simulink library "ifo_new"  (Simulink 8.1)
settings: Solver=ode45  StartTime=0.0  StopTime=10.0  RelTol=1e-3
libraries: hmi x1, gaps x1, ttc x1, sft x1, veh x1, veh_new x1
settings Model: Creator=xsellart  LastModifiedBy=tescamilla

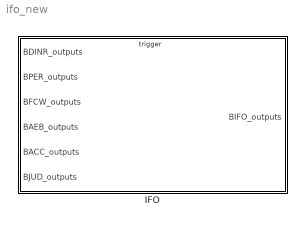
== system ifo_new ==
  IFO : Subsystem

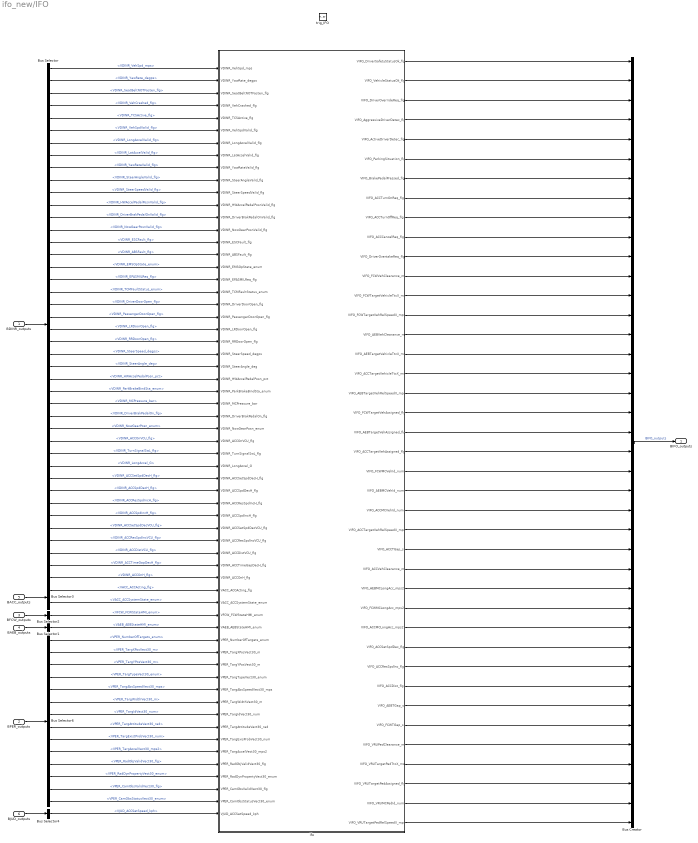
== system ifo_new/IFO ==
  BDINR_outputs : Inport  OutDataTypeStr=Bus: BDINR_outputs
  BPER_outputs : Inport  Port=2  OutDataTypeStr=Bus: BPER_outputs
  BFCW_outputs : Inport  Port=3  OutDataTypeStr=Bus: BFCW_outputs
  BAEB_outputs : Inport  Port=4  OutDataTypeStr=Bus: BAEB_outputs
  BACC_outputs : Inport  Port=5  OutDataTypeStr=Bus: BACC_outputs
  BJUD_outputs : Inport  Port=6  OutDataTypeStr=Bus: BJUD_outputs
  trig_IFO : TriggerPort  TriggerType=function-call
      settings: AttributesFormatString=State = %<StatesWhenEnabling>
  Bus Creator : BusCreator  Inputs=40  OutDataTypeStr=Bus: BIFO_outputs
  Bus Selector : BusSelector  OutputSignals=VDINR_VehSpd_mps,VDINR_YawRate_degps,VDINR_SeatBeltNOTFasten_flg,VDINR_VehCrashed_flg,VDINR_TCSActive_flg,VDINR_VehSpdValid_flg,VDINR_LongAccelValid_flg,VDINR_LatAccelValid_flg,VDINR_YawRateValid_flg,VDINR_SteerAngleValid_flg,VDINR_SteerSpeedValid_flg,VDINR_HWAccelPedalPosnValid_flg,VDINR_DriverBrakPedalOnValid_flg,VDINR_NowGearPosnValid_flg,VDINR_ESCFault_flg,VDINR_ABSFault_flg,VDINR_EMSOpState_enum,VDINR_EPASMILReq_flg,VDINR_TCMFaultStatus_enum,VDINR_DriverDoorOpen_flg,VDINR_PassengerDoorOpen_flg,VDINR_LRDoorOpen_flg,VDINR_RRDoorOpen_flg,VDINR_SteerSpeed_degps,VDINR_SteerAngle_deg,VDINR_HWAccelPedalPosn_pct,VDINR_ParkBrakeBindSta_enum,VDINR_MCPressure_bar,VDINR_DriverBrakPedalOn_flg,VDINR_NowGearPosn_enum,VDINR_ACCOnVCU_flg,VDINR_TurnSignalSwL_flg,VDINR_LongAccel_G,VDINR_ACCSetSpdDecH_flg,VDINR_ACCSpdDecH_flg,VDINR_ACCResSpdIncH_flg,VDINR_ACCSpdIncH_flg,VDINR_ACCSetSpdDecVCU_flg,VDINR_ACCResSpdIncVCU_flg,VDINR_ACCDistVCU_flg,VDINR_ACCTimeGapDecH_flg,VDINR_ACCOnH_flg
  Bus Selector1 : BusSelector  OutputSignals=VAEB_AEBStateHMI_enum
  Bus Selector2 : BusSelector  OutputSignals=VFCW_FCWStateHMI_enum
  Bus Selector3 : BusSelector  OutputSignals=VACC_ACCActing_flg,VACC_ACCSystemState_enum
  Bus Selector4 : BusSelector  OutputSignals=VJUD_ACCSetSpeed_kph
  Bus Selector6 : BusSelector  OutputSignals=VPER_NumberOfTargets_enum,VPER_TargXPosVect30_m,VPER_TargYPosVect30_m,VPER_TargTypeVect30_enum,VPER_TargAbsSpeedVect30_mps,VPER_TargWidthVect30_m,VPER_TargIdVect30_num,VPER_TargAttitudeVect30_rad,VPER_TargExistProbVect30_num,VPER_TargAccelVect30_mps2,VPER_RadObjValidVect30_flg,VPER_RadDynPropertyVect30_enum,VPER_CamObsValidVect30_flg,VPER_CamObsStatusVect30_enum
  ifo : Subsystem
  BIFO_outputs : Outport  OutDataTypeStr=Bus: BIFO_outputs
  wires:
  ifo/26(VIFO_ACCTGap_s) -> Bus Creator/26
  ifo/25(VIFO_ACCTargetVehRelSpeedX_mps) -> Bus Creator/25
  ifo/24(VIFO_ACCMCVehId_num) -> Bus Creator/24
  ifo/23(VIFO_AEBMCVehId_num) -> Bus Creator/23
  ifo/22(VIFO_FCWMCVehId_num) -> Bus Creator/22
  ifo/20(VIFO_AEBTargetVehAssigned_flg) -> Bus Creator/20
  ifo/18(VIFO_AEBTargetVehRelSpeedX_mps) -> Bus Creator/18
  ifo/16(VIFO_AEBTargetVehicleTtcX_ms) -> Bus Creator/16
  ifo/15(VIFO_AEBVehClearance_m) -> Bus Creator/15
  ifo/14(VIFO_FCWTargetVehRelSpeedX_mps) -> Bus Creator/14
  ifo/13(VIFO_FCWTargetVehicleTtcX_ms) -> Bus Creator/13
  ifo/12(VIFO_FCWVehClearance_m) -> Bus Creator/12
  ifo/10(VIFO_ACCCancelReq_flg) -> Bus Creator/10
  ifo/8(VIFO_ACCTurnOnReq_flg) -> Bus Creator/8
  ifo/9(VIFO_ACCTurnOffReq_flg) -> Bus Creator/9
  BDINR_outputs/1 -> Bus Selector/1
  BFCW_outputs/1 -> Bus Selector2/1
  BPER_outputs/1 -> Bus Selector6/1
  Bus Creator/1 -> BIFO_outputs/1  "BIFO_outputs"
  ifo/5(VIFO_ActiveDriverDetec_flg) -> Bus Creator/5
  ifo/4(VIFO_AggressiveDriverDetec_flg) -> Bus Creator/4
  ifo/7(VIFO_BrakePedalPressed_flg) -> Bus Creator/7
  ifo/6(VIFO_ParkingSituation_flg) -> Bus Creator/6
  ifo/1(VIFO_DriverSafetyStatusOk_flg) -> Bus Creator/1
  ifo/3(VIFO_DriverOverrideReq_flg) -> Bus Creator/3
  ifo/2(VIFO_VehicleStatusOk_flg) -> Bus Creator/2
  BAEB_outputs/1 -> Bus Selector1/1
  ifo/27(VIFO_ACCVehClearance_m) -> Bus Creator/27
  ifo/11(VIFO_DriverOvertakeReq_flg) -> Bus Creator/11
  Bus Selector/19 -> ifo/19(VDINR_TCMFaultStatus_enum)  "<VDINR_TCMFaultStatus_enum>"
  Bus Selector/21 -> ifo/21(VDINR_PassengerDoorOpen_flg)  "<VDINR_PassengerDoorOpen_flg>"
  Bus Selector/13 -> ifo/13(VDINR_DriverBrakPedalOnValid_flg)  "<VDINR_DriverBrakPedalOnValid_flg>"
  Bus Selector/11 -> ifo/11(VDINR_SteerSpeedValid_flg)  "<VDINR_SteerSpeedValid_flg>"
  Bus Selector/17 -> ifo/17(VDINR_EMSOpState_enum)  "<VDINR_EMSOpState_enum>"
  Bus Selector/12 -> ifo/12(VDINR_HWAccelPedalPosnValid_flg)  "<VDINR_HWAccelPedalPosnValid_flg>"
  Bus Selector/14 -> ifo/14(VDINR_NowGearPosnValid_flg)  "<VDINR_NowGearPosnValid_flg>"
  Bus Selector/18 -> ifo/18(VDINR_EPASMILReq_flg)  "<VDINR_EPASMILReq_flg>"
  Bus Selector/16 -> ifo/16(VDINR_ABSFault_flg)  "<VDINR_ABSFault_flg>"
  Bus Selector/8 -> ifo/8(VDINR_LatAccelValid_flg)  "<VDINR_LatAccelValid_flg>"
  Bus Selector/20 -> ifo/20(VDINR_DriverDoorOpen_flg)  "<VDINR_DriverDoorOpen_flg>"
  Bus Selector/9 -> ifo/9(VDINR_YawRateValid_flg)  "<VDINR_YawRateValid_flg>"
  Bus Selector/15 -> ifo/15(VDINR_ESCFault_flg)  "<VDINR_ESCFault_flg>"
  Bus Selector/10 -> ifo/10(VDINR_SteerAngleValid_flg)  "<VDINR_SteerAngleValid_flg>"
  Bus Selector/22 -> ifo/22(VDINR_LRDoorOpen_flg)  "<VDINR_LRDoorOpen_flg>"
  Bus Selector/23 -> ifo/23(VDINR_RRDoorOpen_flg)  "<VDINR_RRDoorOpen_flg>"
  Bus Selector/3 -> ifo/3(VDINR_SeatBeltNOTFasten_flg)  "<VDINR_SeatBeltNOTFasten_flg>"
  Bus Selector/6 -> ifo/6(VDINR_VehSpdValid_flg)  "<VDINR_VehSpdValid_flg>"
  Bus Selector/24 -> ifo/24(VDINR_SteerSpeed_degps)  "<VDINR_SteerSpeed_degps>"
  Bus Selector/2 -> ifo/2(VDINR_YawRate_degps)  "<VDINR_YawRate_degps>"
  Bus Selector/4 -> ifo/4(VDINR_VehCrashed_flg)  "<VDINR_VehCrashed_flg>"
  Bus Selector/1 -> ifo/1(VDINR_VehSpd_mps)  "<VDINR_VehSpd_mps>"
  Bus Selector/7 -> ifo/7(VDINR_LongAccelValid_flg)  "<VDINR_LongAccelValid_flg>"
  Bus Selector/5 -> ifo/5(VDINR_TCSActive_flg)  "<VDINR_TCSActive_flg>"
  Bus Selector/30 -> ifo/30(VDINR_NowGearPosn_enum)  "<VDINR_NowGearPosn_enum>"
  Bus Selector/29 -> ifo/29(VDINR_DriverBrakPedalOn_flg)  "<VDINR_DriverBrakPedalOn_flg>"
  Bus Selector/28 -> ifo/28(VDINR_MCPressure_bar)  "<VDINR_MCPressure_bar>"
  Bus Selector/27 -> ifo/27(VDINR_ParkBrakeBindSta_enum)  "<VDINR_ParkBrakeBindSta_enum>"
  Bus Selector/26 -> ifo/26(VDINR_HWAccelPedalPosn_pct)  "<VDINR_HWAccelPedalPosn_pct>"
  Bus Selector/25 -> ifo/25(VDINR_SteerAngle_deg)  "<VDINR_SteerAngle_deg>"
  BACC_outputs/1 -> Bus Selector3/1
  Bus Selector1/1 -> ifo/46(VAEB_AEBStateHMI_enum)  "<VAEB_AEBStateHMI_enum>"
  Bus Selector2/1 -> ifo/45(VFCW_FCWStateHMI_enum)  "<VFCW_FCWStateHMI_enum>"
  Bus Selector3/1 -> ifo/43(VACC_ACCActing_flg)  "<VACC_ACCActing_flg>"
  Bus Selector3/2 -> ifo/44(VACC_ACCSystemState_enum)  "<VACC_ACCSystemState_enum>"
  Bus Selector/32 -> ifo/32(VDINR_TurnSignalSwL_flg)  "<VDINR_TurnSignalSwL_flg>"
  Bus Selector6/1 -> ifo/47(VPER_NumberOfTargets_enum)  "<VPER_NumberOfTargets_enum>"
  Bus Selector6/2 -> ifo/48(VPER_TargXPosVect30_m)  "<VPER_TargXPosVect30_m>"
  Bus Selector6/3 -> ifo/49(VPER_TargYPosVect30_m)  "<VPER_TargYPosVect30_m>"
  Bus Selector6/4 -> ifo/50(VPER_TargTypeVect30_enum)  "<VPER_TargTypeVect30_enum>"
  Bus Selector6/9 -> ifo/55(VPER_TargExisProbVect30_num)  "<VPER_TargExistProbVect30_num>"
  Bus Selector6/6 -> ifo/52(VPER_TargWidthVect30_m)  "<VPER_TargWidthVect30_m>"
  Bus Selector6/7 -> ifo/53(VPER_TargIdVect30_num)  "<VPER_TargIdVect30_num>"
  Bus Selector6/8 -> ifo/54(VPER_TargAttitudeVect30_rad)  "<VPER_TargAttitudeVect30_rad>"
  Bus Selector6/5 -> ifo/51(VPER_TargAbsSpeedVect30_mps)  "<VPER_TargAbsSpeedVect30_mps>"
  BJUD_outputs/1 -> Bus Selector4/1
  Bus Selector4/1 -> ifo/61(VJUD_ACCSetSpeed_kph)  "<VJUD_ACCSetSpeed_kph>"
  Bus Selector/31 -> ifo/31(VDINR_ACCOnVCU_flg)  "<VDINR_ACCOnVCU_flg>"
  Bus Selector/33 -> ifo/33(VDINR_LongAccel_G)  "<VDINR_LongAccel_G>"
  ifo/28(VIFO_AEBMCLongAcc_mps2) -> Bus Creator/28
  ifo/30(VIFO_ACCMCLongAcc_mps2) -> Bus Creator/30
  ifo/29(VIFO_FCWMCLongAcc_mps2) -> Bus Creator/29
  Bus Selector6/11 -> ifo/57(VPER_RadObjValidVect30_flg)  "<VPER_RadObjValidVect30_flg>"
  Bus Selector6/12 -> ifo/58(VPER_RadDynPropertyVect30_enum)  "<VPER_RadDynPropertyVect30_enum>"
  Bus Selector6/10 -> ifo/56(VPER_TargAccelVect30_mps2)  "<VPER_TargAccelVect30_mps2>"
  Bus Selector6/14 -> ifo/60(VPER_CamObsStatusVect30_enum)  "<VPER_CamObsStatusVect30_enum>"
  Bus Selector6/13 -> ifo/59(VPER_CamObsValidVect30_flg)  "<VPER_CamObsValidVect30_flg>"
  ifo/17(VIFO_ACCTargetVehicleTtcX_ms) -> Bus Creator/17
  ifo/21(VIFO_ACCTargetVehAssigned_flg) -> Bus Creator/21
  ifo/19(VIFO_FCWTargetVehAssigned_flg) -> Bus Creator/19
  ifo/32(VIFO_ACCResSpdInc_flg) -> Bus Creator/32
  ifo/33(VIFO_ACCDist_flg) -> Bus Creator/33
  ifo/31(VIFO_ACCSetSpdDec_flg) -> Bus Creator/31
  Bus Selector/34 -> ifo/34(VDINR_ACCSetSpdDecH_flg)  "<VDINR_ACCSetSpdDecH_flg>"
  Bus Selector/35 -> ifo/35(VDINR_ACCSpdDecH_flg)  "<VDINR_ACCSpdDecH_flg>"
  Bus Selector/36 -> ifo/36(VDINR_ACCResSpdIncH_flg)  "<VDINR_ACCResSpdIncH_flg>"
  Bus Selector/37 -> ifo/37(VDINR_ACCSpdIncH_flg)  "<VDINR_ACCSpdIncH_flg>"
  Bus Selector/39 -> ifo/39(VDINR_ACCResSpdIncVCU_flg)  "<VDINR_ACCResSpdIncVCU_flg>"
  Bus Selector/38 -> ifo/38(VDINR_ACCSetSpdDecVCU_flg)  "<VDINR_ACCSetSpdDecVCU_flg>"
  Bus Selector/42 -> ifo/42(VDINR_ACCOnH_flg)  "<VDINR_ACCOnH_flg>"
  Bus Selector/41 -> ifo/41(VDINR_ACCTimeGapDecH_flg)  "<VDINR_ACCTimeGapDecH_flg>"
  Bus Selector/40 -> ifo/40(VDINR_ACCDistVCU_flg)  "<VDINR_ACCDistVCU_flg>"
  ifo/34(VIFO_AEBTGap_s) -> Bus Creator/34
  ifo/35(VIFO_FCWTGap_s) -> Bus Creator/35
  ifo/38(VIFO_VRUTargetPedAssigned_flg) -> Bus Creator/38
  ifo/36(VIFO_VRUPedClearance_m) -> Bus Creator/36
  ifo/39(VIFO_VRUMCPedId_num) -> Bus Creator/39
  ifo/37(VIFO_VRUTargetPedTtcX_ms) -> Bus Creator/37
  ifo/40(VIFO_VRUTargetPedRelSpeedX_mps) -> Bus Creator/40

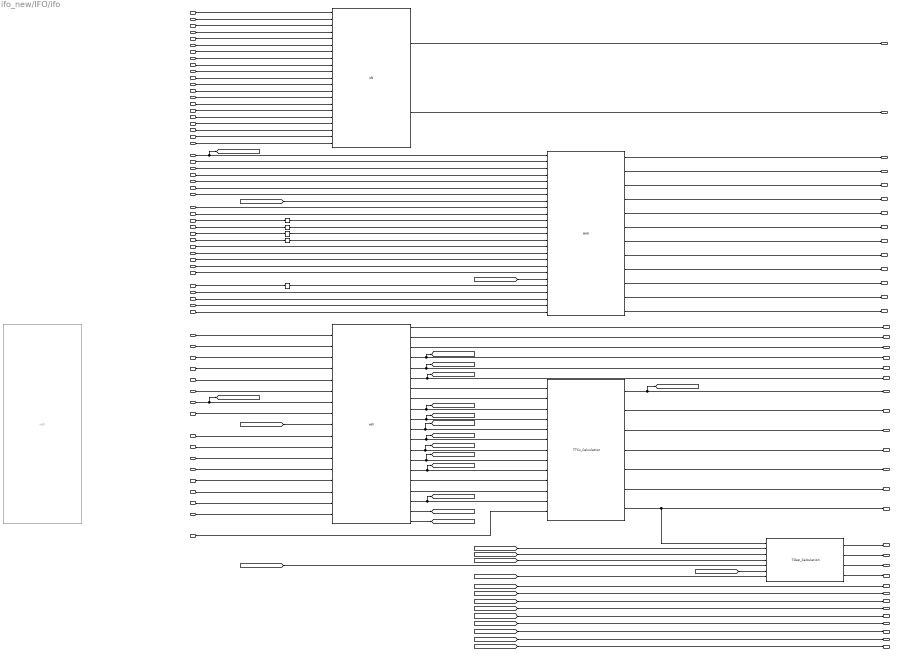
== system ifo_new/IFO/ifo ==
  VDINR_VehSpd_mps : Inport
  VDINR_YawRate_degps : Inport  Port=2
  VDINR_SeatBeltNOTFasten_flg : Inport  Port=3
  VDINR_VehCrashed_flg : Inport  Port=4
  VDINR_TCSActive_flg : Inport  Port=5
  VDINR_VehSpdValid_flg : Inport  Port=6
  VDINR_LongAccelValid_flg : Inport  Port=7
  VDINR_LatAccelValid_flg : Inport  Port=8
  VDINR_YawRateValid_flg : Inport  Port=9
  VDINR_SteerAngleValid_flg : Inport  Port=10
  VDINR_SteerSpeedValid_flg : Inport  Port=11
  VDINR_HWAccelPedalPosnValid_flg : Inport  Port=12
  VDINR_DriverBrakPedalOnValid_flg : Inport  Port=13
  VDINR_NowGearPosnValid_flg : Inport  Port=14
  VDINR_ESCFault_flg : Inport  Port=15
  VDINR_ABSFault_flg : Inport  Port=16
  VDINR_EMSOpState_enum : Inport  Port=17
  VDINR_EPASMILReq_flg : Inport  Port=18
  VDINR_TCMFaultStatus_enum : Inport  Port=19
  VDINR_DriverDoorOpen_flg : Inport  Port=20
  VDINR_PassengerDoorOpen_flg : Inport  Port=21
  VDINR_LRDoorOpen_flg : Inport  Port=22
  VDINR_RRDoorOpen_flg : Inport  Port=23
  VDINR_SteerSpeed_degps : Inport  Port=24
  VDINR_SteerAngle_deg : Inport  Port=25
  VDINR_HWAccelPedalPosn_pct : Inport  Port=26
  VDINR_ParkBrakeBindSta_enum : Inport  Port=27
  VDINR_MCPressure_bar : Inport  Port=28
  VDINR_DriverBrakPedalOn_flg : Inport  Port=29
  VDINR_NowGearPosn_enum : Inport  Port=30
  VDINR_ACCOnVCU_flg : Inport  Port=31
  VDINR_TurnSignalSwL_flg : Inport  Port=32
  VDINR_LongAccel_G : Inport  Port=33
  VDINR_ACCSetSpdDecH_flg : Inport  Port=34
  VDINR_ACCSpdDecH_flg : Inport  Port=35
  VDINR_ACCResSpdIncH_flg : Inport  Port=36
  VDINR_ACCSpdIncH_flg : Inport  Port=37
  VDINR_ACCSetSpdDecVCU_flg : Inport  Port=38
  VDINR_ACCResSpdIncVCU_flg : Inport  Port=39
  VDINR_ACCDistVCU_flg : Inport  Port=40
  VDINR_ACCTimeGapDecH_flg : Inport  Port=41
  VDINR_ACCOnH_flg : Inport  Port=42
  VACC_ACCActing_flg : Inport  Port=43
  VACC_ACCSystemState_enum : Inport  Port=44
  VFCW_FCWStateHMI_enum : Inport  Port=45
  VAEB_AEBStateHMI_enum : Inport  Port=46
  VPER_NumberOfTargets_enum : Inport  Port=47
  VPER_TargXPosVect30_m : Inport  Port=48
  VPER_TargYPosVect30_m : Inport  Port=49
  VPER_TargTypeVect30_enum : Inport  Port=50
  VPER_TargAbsSpeedVect30_mps : Inport  Port=51
  VPER_TargWidthVect30_m : Inport  Port=52
  VPER_TargIdVect30_num : Inport  Port=53
  VPER_TargAttitudeVect30_rad : Inport  Port=54
  VPER_TargExisProbVect30_num : Inport  Port=55
  VPER_TargAccelVect30_mps2 : Inport  Port=56
  VPER_RadObjValidVect30_flg : Inport  Port=57
  VPER_RadDynPropertyVect30_enum : Inport  Port=58
  VPER_CamObsValidVect30_flg : Inport  Port=59
  VPER_CamObsStatusVect30_enum : Inport  Port=60
  VJUD_ACCSetSpeed_kph : Inport  Port=61
  Delay{,1..4} (5 alike) : Delay  DelayLength=1  InitialCondition=0
  HMI : hmi/HMI
  TGap_Calculation : gaps/TGap_Calculation
  TTCx_Calculation : ttc/TTCx_Calculation
  sft : sft/sft
  veh : veh/veh  Commented=on
  veh1 : veh_new/veh
  VIFO_DriverSafetyStatusOk_flg : Outport
  VIFO_VehicleStatusOk_flg : Outport  Port=2
  VIFO_DriverOverrideReq_flg : Outport  Port=3
  VIFO_AggressiveDriverDetec_flg : Outport  Port=4
  VIFO_ActiveDriverDetec_flg : Outport  Port=5
  VIFO_ParkingSituation_flg : Outport  Port=6
  VIFO_BrakePedalPressed_flg : Outport  Port=7
  VIFO_ACCTurnOnReq_flg : Outport  Port=8
  VIFO_ACCTurnOffReq_flg : Outport  Port=9
  VIFO_ACCCancelReq_flg : Outport  Port=10
  VIFO_DriverOvertakeReq_flg : Outport  Port=11
  VIFO_FCWVehClearance_m : Outport  Port=12
  VIFO_FCWTargetVehicleTtcX_ms : Outport  Port=13
  VIFO_FCWTargetVehRelSpeedX_mps : Outport  Port=14
  VIFO_AEBVehClearance_m : Outport  Port=15
  VIFO_AEBTargetVehicleTtcX_ms : Outport  Port=16
  VIFO_ACCTargetVehicleTtcX_ms : Outport  Port=17
  VIFO_AEBTargetVehRelSpeedX_mps : Outport  Port=18
  VIFO_FCWTargetVehAssigned_flg : Outport  Port=19
  VIFO_AEBTargetVehAssigned_flg : Outport  Port=20
  VIFO_ACCTargetVehAssigned_flg : Outport  Port=21
  VIFO_FCWMCVehId_num : Outport  Port=22
  VIFO_AEBMCVehId_num : Outport  Port=23
  VIFO_ACCMCVehId_num : Outport  Port=24
  VIFO_ACCTargetVehRelSpeedX_mps : Outport  Port=25
  VIFO_ACCTGap_s : Outport  Port=26
  VIFO_ACCVehClearance_m : Outport  Port=27
  VIFO_AEBMCLongAcc_mps2 : Outport  Port=28
  VIFO_FCWMCLongAcc_mps2 : Outport  Port=29
  VIFO_ACCMCLongAcc_mps2 : Outport  Port=30
  VIFO_ACCSetSpdDec_flg : Outport  Port=31
  VIFO_ACCResSpdInc_flg : Outport  Port=32
  VIFO_ACCDist_flg : Outport  Port=33
  VIFO_AEBTGap_s : Outport  Port=34
  VIFO_FCWTGap_s : Outport  Port=35
  VIFO_VRUPedClearance_m : Outport  Port=36
  VIFO_VRUTargetPedTtcX_ms : Outport  Port=37
  VIFO_VRUTargetPedAssigned_flg : Outport  Port=38
  VIFO_VRUMCPedId_num : Outport  Port=39
  VIFO_VRUTargetPedRelSpeedX_mps : Outport  Port=40
  wires:
  [VIFO_ACCMCLongAcc_mps2] -> VIFO_ACCMCLongAcc_mps2/1
  [VIFO_ACCTargetVehRelSpeedX_mps] -> VIFO_ACCTargetVehRelSpeedX_mps/1
  veh1/6 -> VIFO_ACCTargetVehAssigned_flg/1, [VIFO_ACCTargetVehAssigned_flg]
  veh1/5 -> VIFO_AEBTargetVehAssigned_flg/1, [VIFO_AEBTargetVehAssigned_flg]
  veh1/4 -> VIFO_FCWTargetVehAssigned_flg/1, [VIFO_FCWTargetVehAssigned_flg]
  veh1/7 -> TTCx_Calculation/1
  veh1/8 -> TTCx_Calculation/2
  veh1/9 -> [VIFO_ACCMCVehXPosition_m], TTCx_Calculation/3
  veh1/10 -> [VIFO_FCWTargetVehRelSpeedX_mps], TTCx_Calculation/4
  veh1/11 -> TTCx_Calculation/5, [VIFO_AEBTargetVehRelSpeedX_mps]
  veh1/12 -> [VIFO_ACCTargetVehRelSpeedX_mps], TTCx_Calculation/6
  veh1/13 -> [VIFO_FCWMCLongAcc_mps2], TTCx_Calculation/7
  veh1/14 -> TTCx_Calculation/8, [VIFO_AEBMCLongAcc_mps2]
  veh1/15 -> [VIFO_ACCMCLongAcc_mps2], TTCx_Calculation/9
  TGap_Calculation/3 -> VIFO_AEBTGap_s/1
  TGap_Calculation/2 -> VIFO_ACCTGap_s/1
  [VDINR_VehSpd_mps] -> TGap_Calculation/5
  [VDINR_VehSpd_mps] -> HMI/8
  HMI/7 -> VIFO_ACCTurnOffReq_flg/1
  veh1/2 -> VIFO_AEBMCVehId_num/1
  veh1/1 -> VIFO_FCWMCVehId_num/1
  sft/2 -> VIFO_VehicleStatusOk_flg/1
  TTCx_Calculation/2 -> VIFO_FCWTargetVehicleTtcX_ms/1
  sft/1 -> VIFO_DriverSafetyStatusOk_flg/1
  HMI/3 -> VIFO_ActiveDriverDetec_flg/1
  HMI/2 -> VIFO_AggressiveDriverDetec_flg/1
  HMI/4 -> VIFO_ParkingSituation_flg/1
  HMI/5 -> VIFO_BrakePedalPressed_flg/1
  TTCx_Calculation/1 -> VIFO_FCWVehClearance_m/1, [VIFO_FCWVehClearance_m]
  HMI/1 -> VIFO_DriverOverrideReq_flg/1
  TTCx_Calculation/3 -> VIFO_AEBTargetVehicleTtcX_ms/1
  VDINR_SteerAngle_deg/1 -> HMI/1, [VDINR_SteerAngle_deg]
  VDINR_SteerSpeed_degps/1 -> HMI/2
  VDINR_HWAccelPedalPosn_pct/1 -> HMI/3
  VDINR_ParkBrakeBindSta_enum/1 -> HMI/4
  VDINR_DriverBrakPedalOn_flg/1 -> HMI/6
  VDINR_NowGearPosn_enum/1 -> HMI/7
  VFCW_FCWStateHMI_enum/1 -> Delay1/1
  VAEB_AEBStateHMI_enum/1 -> Delay/1
  VDINR_EPASMILReq_flg/1 -> sft/16
  VDINR_TCMFaultStatus_enum/1 -> sft/17
  VDINR_EMSOpState_enum/1 -> sft/15
  VDINR_ABSFault_flg/1 -> sft/14
  VDINR_DriverDoorOpen_flg/1 -> sft/18
  VDINR_PassengerDoorOpen_flg/1 -> sft/19
  VDINR_ESCFault_flg/1 -> sft/13
  VDINR_LRDoorOpen_flg/1 -> sft/20
  VDINR_NowGearPosnValid_flg/1 -> sft/12
  VDINR_DriverBrakPedalOnValid_flg/1 -> sft/11
  VDINR_RRDoorOpen_flg/1 -> sft/21
  VDINR_HWAccelPedalPosnValid_flg/1 -> sft/10
  VDINR_SteerSpeedValid_flg/1 -> sft/9
  VDINR_SteerAngleValid_flg/1 -> sft/8
  VDINR_YawRateValid_flg/1 -> sft/7
  VDINR_LatAccelValid_flg/1 -> sft/6
  VDINR_LongAccelValid_flg/1 -> sft/5
  VDINR_VehSpdValid_flg/1 -> sft/4
  VDINR_TCSActive_flg/1 -> sft/3
  VDINR_VehCrashed_flg/1 -> sft/2
  VDINR_SeatBeltNOTFasten_flg/1 -> sft/1
  VDINR_VehSpd_mps/1 -> veh1/7, [VDINR_VehSpd_mps]
  VPER_TargAbsSpeedVect30_mps/1 -> veh1/5
  VPER_TargTypeVect30_enum/1 -> veh1/4
  VPER_TargWidthVect30_m/1 -> veh1/6
  VPER_TargXPosVect30_m/1 -> veh1/2
  VPER_TargYPosVect30_m/1 -> veh1/3
  VDINR_YawRate_degps/1 -> veh1/8
  VPER_NumberOfTargets_enum/1 -> veh1/1
  [VDINR_SteerAngle_deg] -> veh1/9
  VPER_TargIdVect30_num/1 -> veh1/10
  VPER_TargAttitudeVect30_rad/1 -> veh1/11
  VPER_TargExisProbVect30_num/1 -> veh1/12
  [VIFO_AEBTargetVehRelSpeedX_mps] -> VIFO_AEBTargetVehRelSpeedX_mps/1
  [VIFO_FCWTargetVehRelSpeedX_mps] -> VIFO_FCWTargetVehRelSpeedX_mps/1
  VDINR_ACCOnVCU_flg/1 -> HMI/9
  VACC_ACCSystemState_enum/1 -> Delay2/1
  HMI/6 -> VIFO_ACCTurnOnReq_flg/1
  HMI/8 -> VIFO_ACCCancelReq_flg/1
  VACC_ACCActing_flg/1 -> Delay3/1
  TGap_Calculation/1 -> VIFO_ACCVehClearance_m/1
  Delay2/1 -> HMI/13  "VACC_ACCSystemStatePrev_enum"
  Delay/1 -> HMI/12  "VAEB_AEBStateHMIPrev_enum"
  Delay1/1 -> HMI/11  "VFCW_FCWStateHMIPrev_enum"
  VDINR_TurnSignalSwL_flg/1 -> HMI/10
  HMI/9 -> VIFO_DriverOvertakeReq_flg/1
  [VIFO_ACCTargetVehAssigned_flg] -> HMI/20
  Delay3/1 -> HMI/14  "VACC_ACCActingPrev_flg"
  VDINR_MCPressure_bar/1 -> HMI/5
  VPER_TargAccelVect30_mps2/1 -> veh1/13
  VPER_RadObjValidVect30_flg/1 -> veh1/14
  VPER_RadDynPropertyVect30_enum/1 -> veh1/15
  VPER_CamObsValidVect30_flg/1 -> veh1/16
  VPER_CamObsStatusVect30_enum/1 -> veh1/17
  VDINR_LongAccel_G/1 -> TTCx_Calculation/13
  veh1/3 -> VIFO_ACCMCVehId_num/1
  [VIFO_AEBMCLongAcc_mps2] -> VIFO_AEBMCLongAcc_mps2/1
  [VIFO_FCWMCLongAcc_mps2] -> VIFO_FCWMCLongAcc_mps2/1
  Delay4/1 -> HMI/21  "VJUD_ACCSetSpeedPrev_kph"
  TTCx_Calculation/4 -> VIFO_ACCTargetVehicleTtcX_ms/1
  HMI/10 -> VIFO_ACCSetSpdDec_flg/1
  HMI/11 -> VIFO_ACCResSpdInc_flg/1
  HMI/12 -> VIFO_ACCDist_flg/1
  VDINR_ACCOnH_flg/1 -> HMI/25
  VDINR_ACCTimeGapDecH_flg/1 -> HMI/24
  VDINR_ACCDistVCU_flg/1 -> HMI/23
  VDINR_ACCSetSpdDecH_flg/1 -> HMI/15
  VDINR_ACCSpdDecH_flg/1 -> HMI/16
  VDINR_ACCSetSpdDecVCU_flg/1 -> HMI/17
  VDINR_ACCResSpdIncVCU_flg/1 -> HMI/22
  VDINR_ACCResSpdIncH_flg/1 -> HMI/18
  VDINR_ACCSpdIncH_flg/1 -> HMI/19
  VJUD_ACCSetSpeed_kph/1 -> Delay4/1
  [VIFO_ACCTargetVehAssigned_flg] -> TGap_Calculation/4
  TGap_Calculation/4 -> VIFO_FCWTGap_s/1
  [VIFO_FCWVehClearance_m] -> TGap_Calculation/6
  [VIFO_ACCMCVehXPosition_m] -> TGap_Calculation/3
  [VIFO_FCWTargetVehAssigned_flg] -> TGap_Calculation/7
  TTCx_Calculation/7 -> TGap_Calculation/1, VIFO_AEBVehClearance_m/1
  [VIFO_AEBTargetVehAssigned_flg] -> TGap_Calculation/2
  TTCx_Calculation/5 -> VIFO_VRUPedClearance_m/1
  TTCx_Calculation/6 -> VIFO_VRUTargetPedTtcX_ms/1
  veh1/16 -> TTCx_Calculation/10
  veh1/17 -> TTCx_Calculation/11
  veh1/18 -> [VIFO_VRUTargetPedRelSpeedX_mps], TTCx_Calculation/12
  [VIFO_VRUMCPedId_num] -> VIFO_VRUMCPedId_num/1
  [VIFO_VRUTargetPedAssigned_flg] -> VIFO_VRUTargetPedAssigned_flg/1
  veh1/19 -> [VIFO_VRUTargetPedAssigned_flg]
  veh1/20 -> [VIFO_VRUMCPedId_num]
  [VIFO_VRUTargetPedRelSpeedX_mps] -> VIFO_VRUTargetPedRelSpeedX_mps/1
